simulink model "PowerTrain_Simulink"  (R2021a)
settings: Solver=ode23tb  StartTime=0.0  StopTime=500  RelTol=1e-3
undefined symbols (not defined in the file): QuadrotorPowerTrainModel_Object, SYS_Object
settings Model: OrderedModelArguments=off  Creator=renkert2  LastModifiedBy=renkert2
settings SolverCC: AlgebraicLoopSolver=TrustRegion
settings DebuggingCC: SFMachineParentedDataDiag=warning

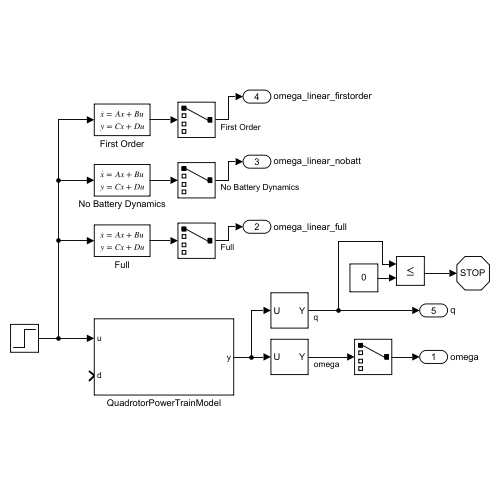
[thumbnail: Simulink's stored preview of the top-level diagram]
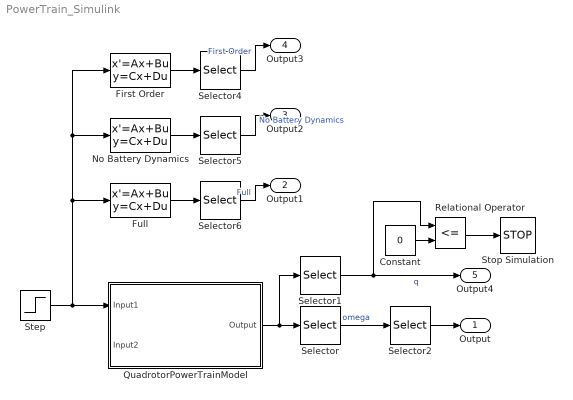
== system PowerTrain_Simulink ==
  Constant : Constant  Value=0
  First Order : StateSpace  A=SYS_Object.PT_Simple.A  B=SYS_Object.PT_Simple.B  C=SYS_Object.PT_Simple.C  D=SYS_Object.PT_Simple.D  InitialCondition=zeros(size(SYS_Object.PT_Simple.A,1),1)
  Full : StateSpace  A=SYS_Object.PT_Full.A  B=SYS_Object.PT_Full.B  C=SYS_Object.PT_Full.C  D=SYS_Object.PT_Full.D  InitialCondition=QuadrotorPowerTrainModel_Object.x0
  No Battery Dynamics : StateSpace  A=SYS_Object.PT_Mod.A  B=SYS_Object.PT_Mod.B  C=SYS_Object.PT_Mod.C  D=SYS_Object.PT_Mod.D  InitialCondition=QuadrotorPowerTrainModel_Object.x0(2:end)
  QuadrotorPowerTrainModel : Subsystem  mask{x_0=QuadrotorPowerTrainModel_Object.x0}
  Relational Operator : RelationalOperator  Operator=<=  OutDataTypeStr=boolean  RndMeth=Simplest
  Selector : Selector  InputPortWidth=QuadrotorPowerTrainModel_Object.Ny  IndexOptions=Index vector (dialog)  Indices=PT_Object.SpeedOutputs_I  OutputSizes=1
  Selector1 : Selector  InputPortWidth=QuadrotorPowerTrainModel_Object.Ny  IndexOptions=Index vector (dialog)  Indices=1  OutputSizes=1
  Selector{2,4..6} (4 alike) : Selector  InputPortWidth=4  IndexOptions=Index vector (dialog)  Indices=[1]  OutputSizes=1
  Step : Step  Before=zeros(4,1)  After=ones(4,1)  SampleTime=0
  Stop Simulation : Stop
  Output : Outport  SignalName=omega
  Output1 : Outport  Port=2  SignalName=omega_linear_full
  Output2 : Outport  Port=3  SignalName=omega_linear_nobatt
  Output3 : Outport  Port=4  SignalName=omega_linear_firstorder
  Output4 : Outport  Port=5  SignalName=q
  wires:
  QuadrotorPowerTrainModel/1(Output) -> Selector1/1, Selector/1
  Selector/1 -> Selector2/1  "omega"
  Selector1/1 -> Relational Operator/1, Output4/1  "q"
  Step/1 -> First Order/1, No Battery Dynamics/1, Full/1, QuadrotorPowerTrainModel/1(Input1)
  First Order/1 -> Selector4/1
  No Battery Dynamics/1 -> Selector5/1
  Full/1 -> Selector6/1
  Selector4/1 -> Output3/1  "First Order"
  Selector5/1 -> Output2/1  "No Battery Dynamics"
  Selector6/1 -> Output1/1  "Full"
  Selector2/1 -> Output/1
  Relational Operator/1 -> Stop Simulation/1
  Constant/1 -> Relational Operator/2

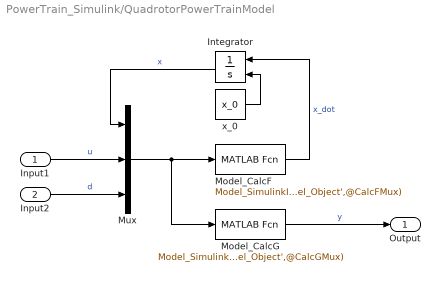
== system PowerTrain_Simulink/QuadrotorPowerTrainModel ==
  Input1 : Inport  PortDimensions=[QuadrotorPowerTrainModel_Object.Nu,1]
  Input2 : Inport  Port=2  PortDimensions=[QuadrotorPowerTrainModel_Object.Nd,1]
  Integrator : Integrator  InitialConditionSource=external
  Model_CalcF : MATLABFcn  MATLABFcn=Model_SimulinkInterpretedFunction(u,'PowerTrain_Simulink','QuadrotorPowerTrainModel_Object',@CalcFMux)  OutputDimensions=QuadrotorPowerTrainModel_Object.Nx
  Model_CalcG : MATLABFcn  MATLABFcn=Model_SimulinkInterpretedFunction(u,'PowerTrain_Simulink','QuadrotorPowerTrainModel_Object',@CalcGMux)  OutputDimensions=QuadrotorPowerTrainModel_Object.Ny
  Mux : Mux  Inputs=3
  x_0 : Constant  Value=x_0  VectorParams1D=off
  Output : Outport
  wires:
  Mux/1 -> Model_CalcF/1, Model_CalcG/1
  Integrator/1 -> Mux/1  "x"
  Input2/1 -> Mux/3  "d"
  x_0/1 -> Integrator/2
  Model_CalcG/1 -> Output/1  "y"
  Input1/1 -> Mux/2  "u"
  Model_CalcF/1 -> Integrator/1  "x_dot"
